simulink model "plant_test"  (R2023b)
settings: Solver=VariableStepAuto  StartTime=0.0  StopTime=t_end  RelTol=1e-3
undefined symbols (not defined in the file): dt, param, sysc, ue, w, x0, xe
libraries: fl_lib x26, nesl_utility x9
(part 3 of 3)

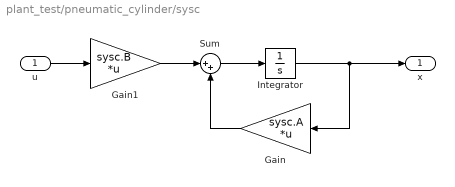
== system plant_test/pneumatic_cylinder/sysc ==
  u : Inport
  Gain : Gain  Gain=sysc.A  Multiplication=Matrix(K*u)
  Gain1 : Gain  Gain=sysc.B  Multiplication=Matrix(K*u)
  Integrator : Integrator  InitialCondition=x0
  Sum : Sum  Inputs=|++
  x : Outport
  wires:
  Sum/1 -> Integrator/1
  u/1 -> Gain1/1
  Gain1/1 -> Sum/1
  Gain/1 -> Sum/2
  Integrator/1 -> x/1, Gain/1

== system plant_test/signal_generator/impulse ==
  Constant1 : Constant  Value=0
  Mux : Mux  Inputs=2
  Step1 : Step  Time=1e-3  Before=1e-3  After=0  SampleTime=0
  target : Outport
  wires:
  Step1/1 -> Mux/1
  Constant1/1 -> Mux/2
  Mux/1 -> target/1

== system plant_test/signal_generator/sine ==
  Constant1 : Constant  Value=0
  Mux : Mux  Inputs=2
  Sine Wave1 : Sin  Amplitude=1e-6  Frequency=w  SampleTime=0
  target : Outport
  wires:
  Sine Wave1/1 -> Mux/1
  Mux/1 -> target/1
  Constant1/1 -> Mux/2

== system plant_test/signal_generator/zero ==
  Constant : Constant  Value=0
  Constant1 : Constant  Value=0
  Mux : Mux  Inputs=2
  target : Outport
  wires:
  Mux/1 -> target/1
  Constant1/1 -> Mux/2
  Constant/1 -> Mux/1

== system plant_test/pneumatic_cylinder/simscape/Vctube ==
  Ta : fl_lib/Thermal/Thermal Sources/Temperature Source  temperature=param.Ta K
  Vctube : fl_lib/Gas/Elements/Constant Volume Chamber (G)  volume=param.Vctube m^3  num_ports=foundation.enum.num_ports.one  area_A=0.01 m^2  area_B=0.01 m^2  area_C=0.01 m^2  area_D=0.01 m^2  p_I_specify=on  p_I_priority=High  p_I=x0(3) Pa  p_I_nominal_specify=off  p_I_nominal_unit=MPa  p_I_nominal_value=1  T_I_specify=off  T_I_priority=High  T_I=293.15 K  T_I_nominal_specify=off  T_I_nominal_unit=K  T_I_nominal_value=1  rho_I_specify=off  rho_I_priority=None  rho_I=1.2 kg/m^3  rho_I_nominal_specify=off  rho_I_nominal_unit=kg/m^3  rho_I_nominal_value=1
      settings: InternalSimscapePortConfiguration="{\"Bottom\":[],\"Left\":[{\"id\":\"A\",\"label\":\"A\",\"type\":\"foundation.gas.gas\"},{\"id\":\"H\",\"label\":\"H\",\"type\":\"foundation.thermal.thermal\"}],\"Right\":[],\"Top\":[]}"
  A : PMIOPort  Side=Left
  B : PMIOPort  Port=2  Side=Right
  connections:
  A/RConn1 -- B/RConn1 -- Vctube/LConn1
  Ta/LConn1 -- Vctube/LConn2

== system plant_test/pneumatic_cylinder/simscape/Vhtube ==
  Ta : fl_lib/Thermal/Thermal Sources/Temperature Source  temperature=param.Ta K
  Vhtube : fl_lib/Gas/Elements/Constant Volume Chamber (G)  volume=param.Vhtube m^3  num_ports=foundation.enum.num_ports.one  area_A=0.01 m^2  area_B=0.01 m^2  area_C=0.01 m^2  area_D=0.01 m^2  p_I_specify=on  p_I_priority=High  p_I=x0(4) Pa  p_I_nominal_specify=off  p_I_nominal_unit=MPa  p_I_nominal_value=1  T_I_specify=off  T_I_priority=High  T_I=293.15 K  T_I_nominal_specify=off  T_I_nominal_unit=K  T_I_nominal_value=1  rho_I_specify=off  rho_I_priority=None  rho_I=1.2 kg/m^3  rho_I_nominal_specify=off  rho_I_nominal_unit=kg/m^3  rho_I_nominal_value=1
      settings: InternalSimscapePortConfiguration="{\"Bottom\":[],\"Left\":[{\"id\":\"A\",\"label\":\"A\",\"type\":\"foundation.gas.gas\"},{\"id\":\"H\",\"label\":\"H\",\"type\":\"foundation.thermal.thermal\"}],\"Right\":[],\"Top\":[]}"
  A : PMIOPort  Side=Left
  B : PMIOPort  Port=2  Side=Right
  connections:
  A/RConn1 -- Vhtube/LConn1 -- B/RConn1
  Ta/LConn1 -- Vhtube/LConn2

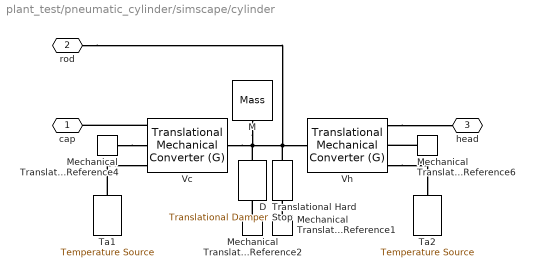
== system plant_test/pneumatic_cylinder/simscape/cylinder ==
  D : fl_lib/Mechanical/Translational Elements/Translational Damper  D=param.D N*s/m  v_specify=off  v_priority=None  v=0 m/s  v_nominal_specify=off  v_nominal_unit=m/s  v_nominal_value=1  f_specify=off  f_priority=None  f=0 N  f_nominal_specify=off  f_nominal_unit=N  f_nominal_value=1
  M : fl_lib/Mechanical/Translational Elements/Mass  mass=param.M kg  num_ports=foundation.enum.numPorts2.one  v_specify=off  v_priority=High  v=0 m/s  v_nominal_specify=off  v_nominal_unit=m/s  v_nominal_value=1  f_specify=off  f_priority=None  f=0 N  f_nominal_specify=off  f_nominal_unit=N  f_nominal_value=1
  Mechanical Translational Reference{1..2,4,6} (4 alike) : fl_lib/Mechanical/Translational Elements/Mechanical Translational Reference
  Ta1 : fl_lib/Thermal/Thermal Sources/Temperature Source  temperature=param.Ta K
  Ta2 : fl_lib/Thermal/Thermal Sources/Temperature Source  temperature=param.Ta K
  Translational Hard Stop : fl_lib/Mechanical/Translational Elements/Translational Hard Stop  upper_bnd=0.5*param.L m  lower_bnd=-0.5*param.L m  model=simscape.enum.hardstop.fulldamped  stiff_up=1e6 N/m  stiff_low=1e6 N/m  D_up=150 N*s/m  D_low=150 N*s/m  transition=0.1 mm  coeff_rest=0.7  v_tol=0.001 m/s  f_tol=0.001 N  v_specify=off  v_priority=None  v=0 m/s  v_nominal_specify=off  v_nominal_unit=m/s  v_nominal_value=1  f_specify=off  f_priority=None  f=0 N  f_nominal_specify=off  f_nominal_unit=N  f_nominal_value=1  x_specify=on  x_priority=High  x=x0(1) m  x_nominal_specify=off  x_nominal_unit=m  x_nominal_value=1  M_specify=off  M_priority=None  M=0
  Vc : fl_lib/Gas/Elements/Translational Mechanical Converter (G)  mech_orientation=foundation.enum.MechOrientationTranslational.Positive  displacement_spec=foundation.enum.DisplacementSpec.Calculate  length_init=x0(1)+0.5*param.L m  interface_area=param.Ac m^2  dead_volume=param.Vc0 m^3  area_A=0.01 m^2  environment_spec=foundation.enum.pressure_spec.atmospheric  environment_pressure=0.101325 MPa  p_I_specify=on  p_I_priority=High  p_I=x0(3) Pa  p_I_nominal_specify=off  p_I_nominal_unit=MPa  p_I_nominal_value=1  T_I_specify=off  T_I_priority=High  T_I=293.15 K  T_I_nominal_specify=off  T_I_nominal_unit=K  T_I_nominal_value=1  rho_I_specify=off  rho_I_priority=None  rho_I=1.2 kg/m^3  rho_I_nominal_specify=off  rho_I_nominal_unit=kg/m^3  rho_I_nominal_value=1
      settings: InternalSimscapePortConfiguration="{\"Bottom\":[],\"Left\":[{\"id\":\"A\",\"label\":\"A\",\"type\":\"foundation.gas.gas\"},{\"id\":\"C\",\"label\":\"C\",\"type\":\"foundation.mechanical.translational.translational\"},{\"id\":\"H\",\"label\":\"H\",\"type\":\"foundation.thermal.thermal\"}],\"Right\":[{\"id\":\"R\",\"label\":\"R\",\"type\":\"foundation.mechanical.translational.translational\"}],\"Top\":[]}"
  Vh : fl_lib/Gas/Elements/Translational Mechanical Converter (G)  mech_orientation=foundation.enum.MechOrientationTranslational.Negative  displacement_spec=foundation.enum.DisplacementSpec.Calculate  length_init=x0(1)-0.5*param.L m  interface_area=param.Ah m^2  dead_volume=param.Vh0 m^3  area_A=0.01 m^2  environment_spec=foundation.enum.pressure_spec.atmospheric  environment_pressure=0.101325 MPa  p_I_specify=on  p_I_priority=High  p_I=x0(4) Pa  p_I_nominal_specify=off  p_I_nominal_unit=MPa  p_I_nominal_value=1  T_I_specify=off  T_I_priority=High  T_I=293.15 K  T_I_nominal_specify=off  T_I_nominal_unit=K  T_I_nominal_value=1  rho_I_specify=off  rho_I_priority=None  rho_I=1.2 kg/m^3  rho_I_nominal_specify=off  rho_I_nominal_unit=kg/m^3  rho_I_nominal_value=1
      settings: InternalSimscapePortConfiguration="{\"Bottom\":[],\"Left\":[{\"id\":\"A\",\"label\":\"A\",\"type\":\"foundation.gas.gas\"},{\"id\":\"C\",\"label\":\"C\",\"type\":\"foundation.mechanical.translational.translational\"},{\"id\":\"H\",\"label\":\"H\",\"type\":\"foundation.thermal.thermal\"}],\"Right\":[{\"id\":\"R\",\"label\":\"R\",\"type\":\"foundation.mechanical.translational.translational\"}],\"Top\":[]}"
  cap : PMIOPort  Side=Left
  rod : PMIOPort  Port=2  Side=Left
  head : PMIOPort  Port=3  Side=Right
  connections:
  Mechanical Translational Reference4/LConn1 -- Vc/LConn2
  Mechanical Translational Reference6/LConn1 -- Vh/LConn2
  Vh/LConn1 -- head/RConn1
  Mechanical Translational Reference2/LConn1 -- D/RConn1
  Vc/RConn1 -- rod/RConn1 -- Translational Hard Stop/LConn1 -- Vh/RConn1 -- M/LConn1 -- D/LConn1
  Mechanical Translational Reference1/LConn1 -- Translational Hard Stop/RConn1
  Vc/LConn1 -- cap/RConn1
  Ta1/LConn1 -- Vc/LConn3
  Vh/LConn3 -- Ta2/LConn1

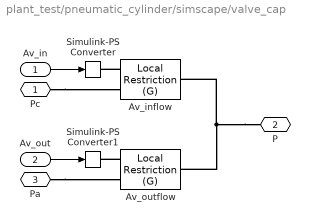
== system plant_test/pneumatic_cylinder/simscape/valve_cap ==
  Av_in : Inport
  Av_out : Inport  Port=2
  Av_inflow : fl_lib/Gas/Elements/Local Restriction (G)  restriction_type=foundation.enum.restriction_type.variable  restriction_area=1e-3 m^2  min_area=eps m^2  max_area=param.Av m^2  area=0.01 m^2  Cd=0.8975  B_lam=0.999
      settings: InternalSimscapePortConfiguration="{\"Bottom\":[],\"Left\":[{\"id\":\"A\",\"label\":\"A\",\"type\":\"foundation.gas.gas\"},{\"id\":\"area_in\",\"label\":\"AR\",\"type\":\"input\"}],\"Right\":[{\"id\":\"B\",\"label\":\"B\",\"type\":\"foundation.gas.gas\"}],\"Top\":[]}"
  Av_outflow : fl_lib/Gas/Elements/Local Restriction (G)  restriction_type=foundation.enum.restriction_type.variable  restriction_area=1e-3 m^2  min_area=eps m^2  max_area=param.Av m^2  area=0.01 m^2  Cd=0.8975  B_lam=0.999
      settings: InternalSimscapePortConfiguration="{\"Bottom\":[],\"Left\":[{\"id\":\"A\",\"label\":\"A\",\"type\":\"foundation.gas.gas\"},{\"id\":\"area_in\",\"label\":\"AR\",\"type\":\"input\"}],\"Right\":[{\"id\":\"B\",\"label\":\"B\",\"type\":\"foundation.gas.gas\"}],\"Top\":[]}"
  Simulink-PS Converter : nesl_utility/Simulink-PS Converter  PhysicalDomain=network_engine_domain  SubClassName=ps_input  LeftPortType=input  RightPortType=output  PseudoPeriodic=off  Frequencies=[]  NoiseDistribution=none  NoiseParameters=[]  Unit=1  AffineConversion=off  FilteringAndDerivatives=provide  SimscapeFilterOrder=1  InputFilterTimeConstant=0.001  UdotUserProvided=0
  Simulink-PS Converter1 : nesl_utility/Simulink-PS Converter  PhysicalDomain=network_engine_domain  SubClassName=ps_input  LeftPortType=input  RightPortType=output  PseudoPeriodic=off  Frequencies=[]  NoiseDistribution=none  NoiseParameters=[]  Unit=1  AffineConversion=off  FilteringAndDerivatives=provide  SimscapeFilterOrder=1  InputFilterTimeConstant=0.001  UdotUserProvided=0
  Pc : PMIOPort  Side=Left
  P : PMIOPort  Port=2  Side=Right
  Pa : PMIOPort  Port=3  Side=Right
  wires:
  Av_in/1 -> Simulink-PS Converter/1
  Av_out/1 -> Simulink-PS Converter1/1
  connections:
  Pc/RConn1 -- Av_inflow/LConn1
  Av_inflow/LConn2 -- Simulink-PS Converter/RConn1
  Pa/RConn1 -- Av_outflow/LConn1
  Av_outflow/LConn2 -- Simulink-PS Converter1/RConn1
  P/RConn1 -- Av_outflow/RConn1 -- Av_inflow/RConn1

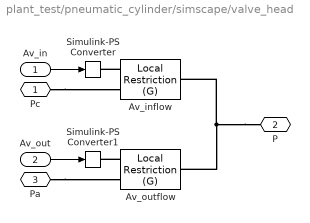
== system plant_test/pneumatic_cylinder/simscape/valve_head ==
  Av_in : Inport
  Av_out : Inport  Port=2
  Av_inflow : fl_lib/Gas/Elements/Local Restriction (G)  restriction_type=foundation.enum.restriction_type.variable  restriction_area=1e-3 m^2  min_area=eps m^2  max_area=param.Av m^2  area=0.01 m^2  Cd=0.8975  B_lam=0.999
      settings: InternalSimscapePortConfiguration="{\"Bottom\":[],\"Left\":[{\"id\":\"A\",\"label\":\"A\",\"type\":\"foundation.gas.gas\"},{\"id\":\"area_in\",\"label\":\"AR\",\"type\":\"input\"}],\"Right\":[{\"id\":\"B\",\"label\":\"B\",\"type\":\"foundation.gas.gas\"}],\"Top\":[]}"
  Av_outflow : fl_lib/Gas/Elements/Local Restriction (G)  restriction_type=foundation.enum.restriction_type.variable  restriction_area=1e-3 m^2  min_area=eps m^2  max_area=param.Av m^2  area=0.01 m^2  Cd=0.8975  B_lam=0.999
      settings: InternalSimscapePortConfiguration="{\"Bottom\":[],\"Left\":[{\"id\":\"A\",\"label\":\"A\",\"type\":\"foundation.gas.gas\"},{\"id\":\"area_in\",\"label\":\"AR\",\"type\":\"input\"}],\"Right\":[{\"id\":\"B\",\"label\":\"B\",\"type\":\"foundation.gas.gas\"}],\"Top\":[]}"
  Simulink-PS Converter : nesl_utility/Simulink-PS Converter  PhysicalDomain=network_engine_domain  SubClassName=ps_input  LeftPortType=input  RightPortType=output  PseudoPeriodic=off  Frequencies=[]  NoiseDistribution=none  NoiseParameters=[]  Unit=1  AffineConversion=off  FilteringAndDerivatives=provide  SimscapeFilterOrder=1  InputFilterTimeConstant=0.001  UdotUserProvided=0
  Simulink-PS Converter1 : nesl_utility/Simulink-PS Converter  PhysicalDomain=network_engine_domain  SubClassName=ps_input  LeftPortType=input  RightPortType=output  PseudoPeriodic=off  Frequencies=[]  NoiseDistribution=none  NoiseParameters=[]  Unit=1  AffineConversion=off  FilteringAndDerivatives=provide  SimscapeFilterOrder=1  InputFilterTimeConstant=0.001  UdotUserProvided=0
  Pc : PMIOPort  Side=Left
  P : PMIOPort  Port=2  Side=Right
  Pa : PMIOPort  Port=3  Side=Right
  wires:
  Av_in/1 -> Simulink-PS Converter/1
  Av_out/1 -> Simulink-PS Converter1/1
  connections:
  Pc/RConn1 -- Av_inflow/LConn1
  Av_inflow/LConn2 -- Simulink-PS Converter/RConn1
  Pa/RConn1 -- Av_outflow/LConn1
  Av_outflow/LConn2 -- Simulink-PS Converter1/RConn1
  P/RConn1 -- Av_outflow/RConn1 -- Av_inflow/RConn1

== matlab function plant_test/pneumatic_cylinder/ode/MATLAB Function ==
  data: x input size=param.xdim; u input size=param.udim; dxdt output size=param.xdim; param parameter
function dxdt = ode(x,u,param)
    dxdt = plant_ode(0,x,u,param);
end

== matlab function plant_test/input_transform/udim==4/valve ==
  data: mu input size=2; x input size=4; Av output size=4; param parameter
function Av = valve(mu,x,param)
    Pa = param.Pa;
    Ps = param.Ps;
    alpha_in = param.alpha_in;
    alpha_out = param.alpha_out;

    Pc = x(3);
    Ph = x(4);
    muc = mu(1);
    muh = mu(2);

    if muc > 0
        Avc = [muc/(alpha_in*phi(Ps,Pc,param));0];
    elseif muc < 0
        Avc = [0;-muc/(alpha_out*phi(Pc,Pa,param))];
    else
        Avc = [0;0];
    end

    if muh > 0
        Avh = [muh/(alpha_in*phi(Ps,Ph,param));0];
    elseif muh < 0
        Avh = [0;-muh/(alpha_out*phi(Ph,Pa,param))];
    else
        Avh = [0;0];
    end

    Av = [Avc;Avh];
end

function ret = phi(P1,P2,param)
    R = param.R;
    Ta = param.Ta;
    k = param.k;
    Pcr = (2/(k + 1))^(k/(k - 1)); % critical pressure ratio (-)
    C1 = sqrt(k*(2/(k + 1))^((k + 1)/(k - 1)));
    C2 = sqrt(2*k/(k - 1));

    if (P2/P1) < Pcr
        ret = C1*(P1/sqrt(R*Ta));
    elseif (P2/P1) < 1
        ret = C2*(P1/sqrt(R*Ta))*(P2/P1)^(1/k)*sqrt(1 - (P2/P1)^((k - 1)/k));
    elseif (P2/P1) < (1/Pcr)
        ret = -C2*(P2/sqrt(R*Ta))*(P1/P2)^(1/k)*sqrt(1 - (P1/P2)^((k - 1)/k));
    else
        ret = -C1*(P2/sqrt(R*Ta));
    end
end
